simulink model "lqr_model"  (R2021a)
settings: Solver=VariableStepAuto  StartTime=0.0  StopTime=20  FixedStep=0.01  RelTol=1e-3
values from neighbouring files (symbols this model uses):
  FF_L = op.inputs(1).u    [trim_boat.m]
  initial_P = op.states(7).x    [trim_boat.m]
  initial_Q = op.states(3).x    [trim_boat.m]
  initial_R = op.states(8).x    [trim_boat.m]
  initial_uspeed = op.states(1).x    [trim_boat.m]
  initial_vspeed = op.states(6).x    [trim_boat.m]
  initial_wspeed = op.states(2).x    [trim_boat.m]
  initial_Z = op.states(5).x    [trim_boat.m]
  rear_alfas = op.inputs(3).u    [trim_boat.m]
  T = op.inputs(4).u    [trim_boat.m]
undefined symbols (not defined in the file or in its folder): ap2, ar2, ay2, bp2, br2, by2, Eff, K
libraries: simulink x4, pid_lib x1, dsparch4 x1
(part 1 of 2)
settings Model: Creator=Basile  LastModifiedBy=simao
settings SolverCC: ConcurrentTasks=on  ZeroCrossAlgorithm=Adaptive  AlgebraicLoopSolver=TrustRegion  PositivePriorityOrder=on
settings DataIOCC: ExternalInput=getinputstruct(op_trim1)  InitialState=getstatestruct(op_trim1)  SaveOutput=off  DSMLogging=off  SaveTime=off  ReturnWorkspaceOutputs=off
settings OptimizationCC: BlockReduction=off  DefaultParameterBehavior=Inlined  UseDivisionForNetSlopeComputation=on  UseFloatMulNetSlope=on  OptimizeBlockIOStorage=off  BufferReuse=off  PassReuseOutputArgsThreshold=0  EfficientFloat2IntCast=on  OptimizeBlockOrder=speed  DifferentSizesBufferReuse=on
settings DebuggingCC: InheritedTsInSrcMsg=none  ParameterTunabilityLossMsg=error  UnconnectedInputMsg=none  UnconnectedOutputMsg=none  UnconnectedLineMsg=none  UniqueDataStoreMsg=error  SFMachineParentedDataDiag=warning  ArithmeticOperatorsInVariantConditions=warning
settings HardwareCC: ProdBitPerLong=64  ProdLongLongMode=on  ProdHWDeviceType=Intel->x86-64 (Linux 64)
settings SFSimCC: SimUseLocalCustomCode=off  MATLABDynamicMemAlloc=off  CustomCodeUndefinedFunction=UseInterfaceOnly
settings RTWCC: Description=Simulink Real-Time  SystemTargetFile=slrealtime.tlc  TemplateMakefile=slrealtime_default_tmf  GenerateReport=on  RTWUseLocalCustomCode=off  Toolchain=Simulink Real-Time Toolchain  BuildConfiguration=Faster Runs  LaunchReport=on  CodeExecutionProfiling=on  TargetLang=C++
settings CodeAppCC: ForceParamTrailComments=on  OperatorAnnotations=on

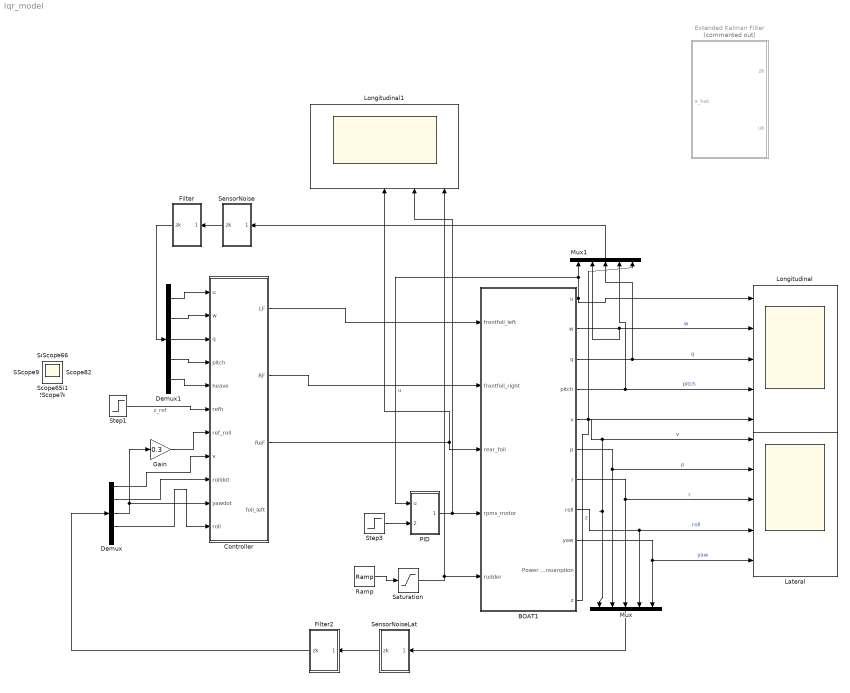
== system lqr_model ==
  BOAT1 : Subsystem
  Controller : Subsystem
  Demux : Demux  Outputs=5
  Demux1 : Demux  Outputs=5
  Extended Kalman Filter : Subsystem  Commented=on
  Filter : Subsystem
  Filter2 : Subsystem
  Gain : Gain  Gain=0.3
  Lateral : Scope  NumInputPorts=5
  Longitudinal : Scope  NumInputPorts=5
  Longitudinal1 : Scope  NumInputPorts=5
  Mux : Mux  Inputs=5
  Mux1 : Mux  Inputs=5
  PID : Subsystem
  Ramp : simulink/Sources/Ramp  slope=15  start=0  InitialOutput=0
  Saturation : Saturate  UpperLimit=0  LowerLimit=0
  SensorNoise : Subsystem
  SensorNoiseLat : Subsystem
  Step1 : Step  Time=0  Before=initial_Z  After=-0.4  SampleTime=0
  Step3 : Step  Time=0  Before=initial_uspeed  After=7  SampleTime=0
  Scope{,1..66} (67 alike) : Scope
  wires:
  BOAT1/2(w) -> Mux1/2, Longitudinal/2  "w"
  BOAT1/3(q) -> Mux1/3, Longitudinal/3  "q"
  BOAT1/5(v) -> Mux/1, Lateral/1  "v"
  BOAT1/6(p) -> Lateral/2, Mux/2  "p"
  BOAT1/8(roll) -> Lateral/4, Mux/4  "roll"
  BOAT1/11(z) -> Mux1/5, Longitudinal/5  "z"
  BOAT1/1(u) -> Longitudinal/1, PID/1(u), Mux1/1  "u"
  BOAT1/7(r) -> Lateral/3, Mux/3  "r"
  Demux1/2 -> Controller/2(w)
  Demux1/3 -> Controller/3(q)
  Demux1/4 -> Controller/4(pitch)
  Demux1/5 -> Controller/5(heave)
  Demux1/1 -> Controller/1(u)
  BOAT1/9(yaw) -> Mux/5, Lateral/5  "yaw"
  BOAT1/4(pitch) -> Mux1/4, Longitudinal/4  "pitch"
  Mux1/1 -> SensorNoise/1(states)
  Step1/1 -> Controller/6(refh)  "z_ref"
  Mux/1 -> SensorNoiseLat/1(states)
  Step3/1 -> PID/2(In2)
  Controller/3(ReF) -> BOAT1/3(rear_foil), Longitudinal1/3
  PID/1(rpms_motor) -> BOAT1/4(rpms_motor), Longitudinal1/4
  SensorNoise/1(zk) -> Filter/1(states)
  SensorNoiseLat/1(zk) -> Filter2/1(states)
  Filter/1(zk) -> Demux1/1
  Filter2/1(zk) -> Demux/1
  Gain/1 -> Controller/7(ref_roll)
  Ramp/1 -> Saturation/1
  Saturation/1 -> BOAT1/5(rudder), Longitudinal1/5
  Demux/2 -> Controller/9(rolldot)
  Demux/3 -> Gain/1, Controller/10(yawdot)
  Demux/4 -> Controller/11(roll)
  Demux/1 -> Controller/8(v)
  Controller/1(LF) -> BOAT1/1(frontfoil_left)
  Controller/2(RF) -> BOAT1/2(frontfoil_right)

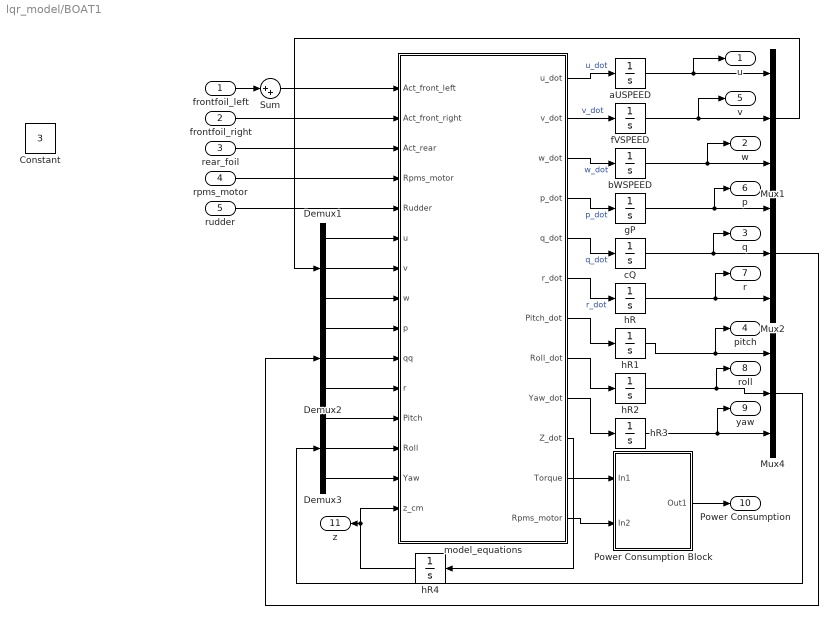
== system lqr_model/BOAT1 ==
  frontfoil_left : Inport
  frontfoil_right : Inport  Port=2
  rear_foil : Inport  Port=3
  rpms_motor : Inport  Port=4
  rudder : Inport  Port=5
  Constant : Constant  Value=3
  Demux1 : Demux  Outputs=3
  Demux2 : Demux  Outputs=3
  Demux3 : Demux  Outputs=3
  Mux1 : Mux  Inputs=3
  Mux2 : Mux  Inputs=3
  Mux4 : Mux  Inputs=3
  Power Consumption Block : Subsystem
  Sum : Sum  Inputs=|++
  aUSPEED : Integrator  InitialCondition=initial_uspeed
  bWSPEED : Integrator  InitialCondition=initial_wspeed
  cQ : Integrator  InitialCondition=initial_Q
  fVSPEED : Integrator  InitialCondition=initial_vspeed
  gP : Integrator  InitialCondition=initial_P
  hR : Integrator  InitialCondition=initial_R
  hR1 : Integrator
  hR2 : Integrator
  hR3 : Integrator
  hR4 : Integrator  InitialCondition=initial_Z
  model_equations : MATLAB Function  TreatAsAtomicUnit=on  VariantControl=Variant1
  u : Outport  VectorParamsAs1DForOutWhenUnconnected=off
  w : Outport  Port=2  VectorParamsAs1DForOutWhenUnconnected=off
  q : Outport  Port=3  VectorParamsAs1DForOutWhenUnconnected=off
  pitch : Outport  Port=4  VectorParamsAs1DForOutWhenUnconnected=off
  v : Outport  Port=5  VectorParamsAs1DForOutWhenUnconnected=off
  p : Outport  Port=6  VectorParamsAs1DForOutWhenUnconnected=off
  r : Outport  Port=7  VectorParamsAs1DForOutWhenUnconnected=off
  roll : Outport  Port=8  VectorParamsAs1DForOutWhenUnconnected=off
  yaw : Outport  Port=9  VectorParamsAs1DForOutWhenUnconnected=off
  Power Consumption : Outport  Port=10  VectorParamsAs1DForOutWhenUnconnected=off
  z : Outport  Port=11  VectorParamsAs1DForOutWhenUnconnected=off
  wires:
  model_equations/6(r_dot) -> hR/1  "r_dot"
  Mux1/1 -> Demux1/1
  model_equations/5(q_dot) -> cQ/1  "q_dot"
  rear_foil/1 -> model_equations/3(Act_rear)
  Demux3/2 -> model_equations/13(Roll)
  Demux2/2 -> model_equations/10(qq)
  Demux2/3 -> model_equations/11(r)
  model_equations/4(p_dot) -> gP/1  "p_dot"
  Demux2/1 -> model_equations/9(p)
  rpms_motor/1 -> model_equations/4("Rpms_motor ")
  Demux3/1 -> model_equations/12(Pitch)
  model_equations/2(v_dot) -> fVSPEED/1  "v_dot"
  Demux1/2 -> model_equations/7(v)
  Mux2/1 -> Demux2/1
  Demux3/3 -> model_equations/14(Yaw)
  model_equations/12(Rpms_motor) -> Power Consumption Block/2(In2)
  Power Consumption Block/1(Out1) -> Power Consumption/1
  model_equations/11(Torque) -> Power Consumption Block/1(In1)
  Demux1/1 -> model_equations/6(u)
  cQ/1 -> q/1, Mux2/2
  hR/1 -> Mux2/3, r/1
  model_equations/3(w_dot) -> bWSPEED/1  "w_dot"
  model_equations/1(u_dot) -> aUSPEED/1  "u_dot"
  gP/1 -> p/1, Mux2/1
  model_equations/7(Pitch_dot) -> hR1/1
  model_equations/8(Roll_dot) -> hR2/1
  model_equations/9(Yaw_dot) -> hR3/1
  hR1/1 -> pitch/1, Mux4/1
  hR2/1 -> roll/1, Mux4/2
  hR3/1 -> yaw/1, Mux4/3
  Mux4/1 -> Demux3/1
  rudder/1 -> model_equations/5(Rudder)
  frontfoil_right/1 -> model_equations/2(Act_front_right)
  frontfoil_left/1 -> Sum/1
  Sum/1 -> model_equations/1(Act_front_left)
  Demux1/3 -> model_equations/8(w)
  fVSPEED/1 -> v/1, Mux1/2
  aUSPEED/1 -> u/1, Mux1/1
  bWSPEED/1 -> w/1, Mux1/3
  model_equations/10(Z_dot) -> hR4/1
  hR4/1 -> model_equations/15(z_cm), z/1

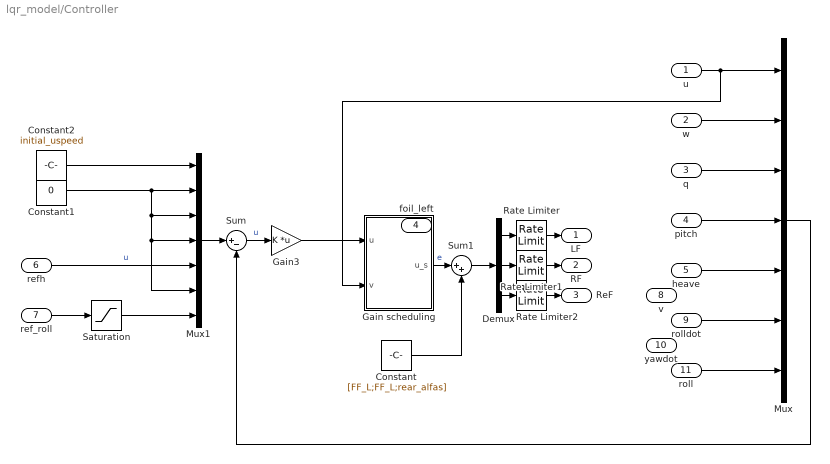
== system lqr_model/Controller ==
  u : Inport
  w : Inport  Port=2
  q : Inport  Port=3
  pitch : Inport  Port=4
  heave : Inport  Port=5
  refh : Inport  Port=6
  ref_roll : Inport  Port=7
  v : Inport  Port=8
  rolldot : Inport  Port=9
  yawdot : Inport  Port=10
  roll : Inport  Port=11
  Constant : Constant  Value=[FF_L;FF_L;rear_alfas]
  Constant1 : Constant  Value=0
  Constant2 : Constant  Value=initial_uspeed
  Demux : Demux  Outputs=3
  Gain scheduling : MATLAB Function  TreatAsAtomicUnit=on
  Gain3 : Gain  Gain=K  Multiplication=Matrix(K*u)
  Mux : Mux  Inputs=7
  Mux1 : Mux  Inputs=7
  Rate Limiter : RateLimiter  RisingSlewLimit=10  FallingSlewLimit=-10  SampleTimeMode=inherited  InitialCondition=FF_L
  Rate Limiter1 : RateLimiter  RisingSlewLimit=10  FallingSlewLimit=-10  SampleTimeMode=inherited  InitialCondition=FF_L
  Rate Limiter2 : RateLimiter  SampleTimeMode=inherited  InitialCondition=rear_alfas
  Saturation : Saturate  UpperLimit=3  LowerLimit=-3
  Sum : Sum  Inputs=|+-
  Sum1 : Sum  Inputs=|++
  LF : Outport  VectorParamsAs1DForOutWhenUnconnected=off
  RF : Outport  Port=2  VectorParamsAs1DForOutWhenUnconnected=off
  ReF : Outport  Port=3  VectorParamsAs1DForOutWhenUnconnected=off
  foil_left : Outport  Port=4  VectorParamsAs1DForOutWhenUnconnected=off
  wires:
  ref_roll/1 -> Saturation/1
  Mux/1 -> Sum/2
  u/1 -> Gain scheduling/2(v), Mux/1
  w/1 -> Mux/2
  q/1 -> Mux/3
  pitch/1 -> Mux/4
  heave/1 -> Mux/5
  rolldot/1 -> Mux/6
  roll/1 -> Mux/7
  Mux1/1 -> Sum/1
  refh/1 -> Mux1/5  "u"
  Sum/1 -> Gain3/1  "u"
  Saturation/1 -> Mux1/7
  Constant1/1 -> Mux1/6, Mux1/4, Mux1/3, Mux1/2
  Constant2/1 -> Mux1/1
  Gain3/1 -> Gain scheduling/1(u)
  Gain scheduling/1(u_s) -> Sum1/1  "e"
  Sum1/1 -> Demux/1
  Constant/1 -> Sum1/2
  Demux/1 -> Rate Limiter/1
  Rate Limiter/1 -> LF/1
  Demux/2 -> Rate Limiter1/1
  Rate Limiter1/1 -> RF/1
  Demux/3 -> Rate Limiter2/1
  Rate Limiter2/1 -> ReF/1

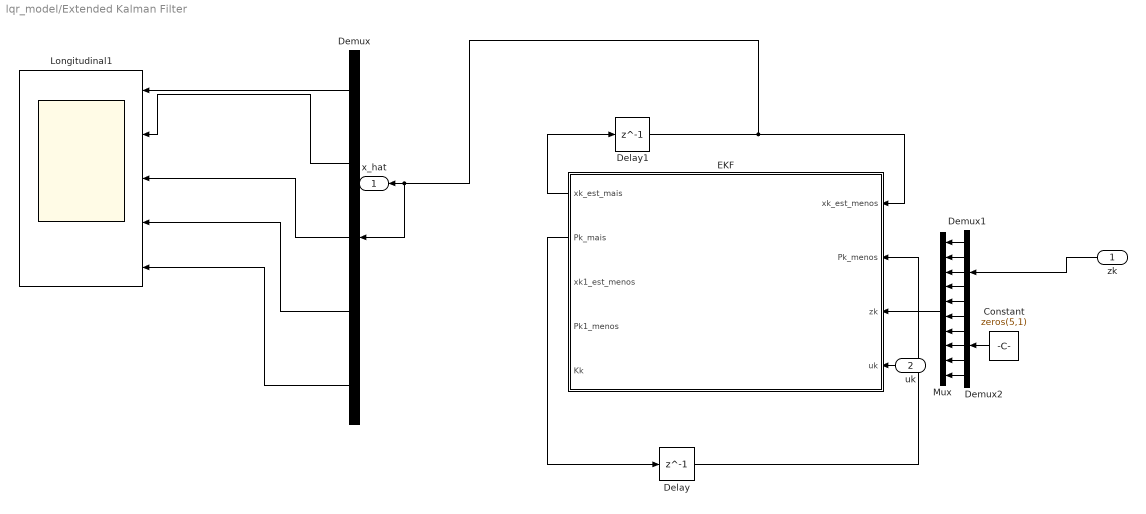
== system lqr_model/Extended Kalman Filter ==
  zk : Inport  PortDimensions=5
  uk : Inport  Port=2  PortDimensions=5
  Constant : Constant  Value=zeros(5,1)
  Delay : Delay  DelayLength=1  InitialCondition=1000*eye(37)  SampleTime=0.02
  Delay1 : Delay  DelayLength=1  InitialCondition=[initial_uspeed;0;0;0;initial_Z;0;0;0;0;0;zeros(27,1)]  SampleTime=0.02
  Demux : Demux  Outputs=5
  Demux1 : Demux  Outputs=5
  Demux2 : Demux  Outputs=5
  EKF : MATLAB Function  TreatAsAtomicUnit=on
  Longitudinal1 : Scope  NumInputPorts=5
  Mux : Mux  Inputs=10
  x_hat : Outport
  wires:
  uk/1 -> EKF/4(uk)
  Delay/1 -> EKF/2(Pk_menos)
  Demux/1 -> Longitudinal1/1
  Demux/2 -> Longitudinal1/2
  Demux/3 -> Longitudinal1/3
  Demux/4 -> Longitudinal1/4
  Demux/5 -> Longitudinal1/5
  Delay1/1 -> Demux/1, x_hat/1, EKF/1(xk_est_menos)
  EKF/2(Pk_mais) -> Delay/1
  EKF/1(xk_est_mais) -> Delay1/1
  zk/1 -> Demux1/1
  Mux/1 -> EKF/3(zk)
  Demux1/1 -> Mux/1
  Demux1/2 -> Mux/2
  Demux1/3 -> Mux/3
  Demux1/4 -> Mux/4
  Demux1/5 -> Mux/5
  Demux2/1 -> Mux/6
  Demux2/2 -> Mux/7
  Demux2/3 -> Mux/8
  Demux2/4 -> Mux/9
  Demux2/5 -> Mux/10
  Constant/1 -> Demux2/1

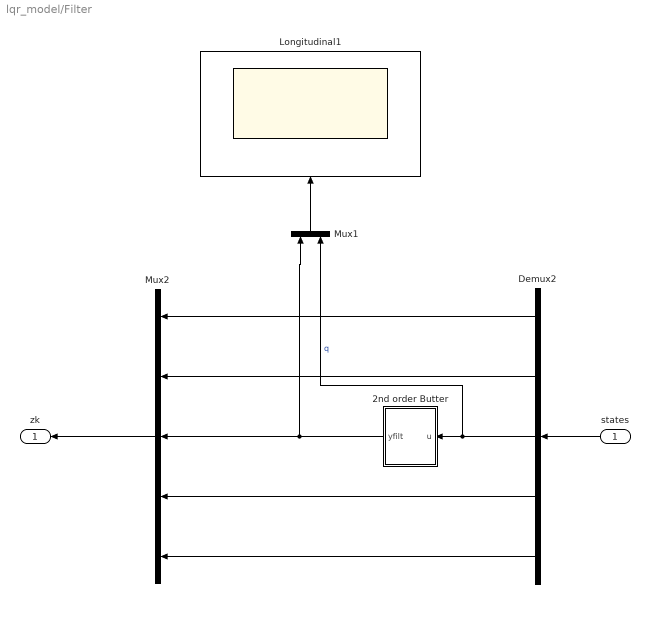
== system lqr_model/Filter ==
  states : Inport
  2nd order Butter : Subsystem
  Demux2 : Demux  Outputs=5
  Longitudinal1 : Scope  NumInputPorts=5
  Mux1 : Mux  Inputs=2
  Mux2 : Mux  Inputs=5
  zk : Outport
  wires:
  states/1 -> Demux2/1
  Mux2/1 -> zk/1
  Demux2/1 -> Mux2/1
  Demux2/2 -> Mux2/2
  Demux2/4 -> Mux2/4
  Demux2/5 -> Mux2/5
  Mux1/1 -> Longitudinal1/3
  2nd order Butter/1(yfilt) -> Mux1/1, Mux2/3
  Demux2/3 -> Mux1/2, 2nd order Butter/1(u)  "q"

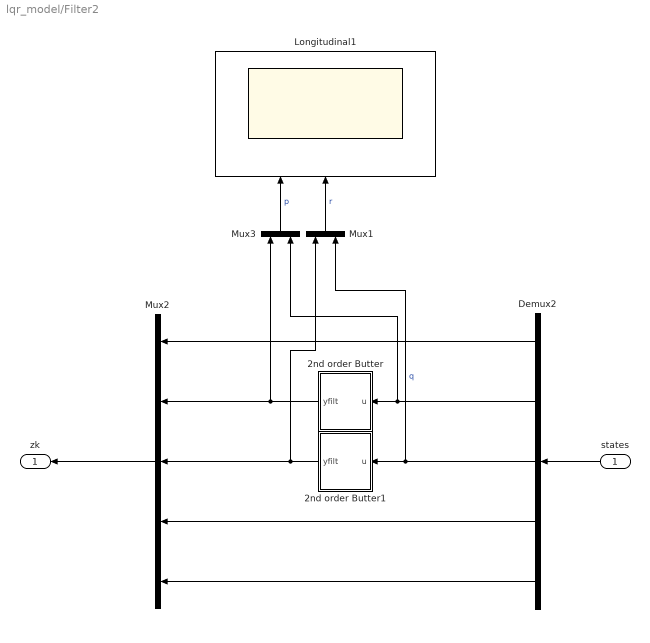
== system lqr_model/Filter2 ==
  states : Inport
  2nd order Butter : Subsystem
  2nd order Butter1 : Subsystem
  Demux2 : Demux  Outputs=5
  Longitudinal1 : Scope  NumInputPorts=5
  Mux1 : Mux  Inputs=2
  Mux2 : Mux  Inputs=5
  Mux3 : Mux  Inputs=2
  zk : Outport
  wires:
  states/1 -> Demux2/1
  Mux2/1 -> zk/1
  Demux2/1 -> Mux2/1
  Demux2/4 -> Mux2/4
  Demux2/5 -> Mux2/5
  Demux2/2 -> Mux3/2, 2nd order Butter/1(u)
  2nd order Butter/1(yfilt) -> Mux3/1, Mux2/2
  2nd order Butter1/1(yfilt) -> Mux1/1, Mux2/3
  Demux2/3 -> Mux1/2, 2nd order Butter1/1(u)  "q"
  Mux1/1 -> Longitudinal1/3  "r"
  Mux3/1 -> Longitudinal1/2  "p"

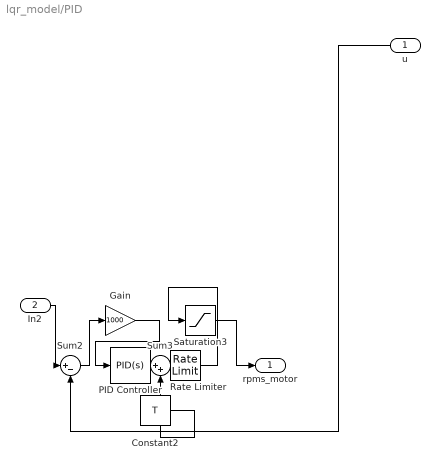
== system lqr_model/PID ==
  u : Inport
  In2 : Inport  Port=2
  Constant2 : Constant  Value=T
  Gain : Gain  Gain=1000
  PID Controller : pid_lib/PID Controller  Controller=PID  Form=Parallel  TimeDomain=Continuous-time  UseExternalTs=off  SampleTime=-1  IntegratorMethod=Forward Euler  FilterMethod=Forward Euler  ControllerParametersSource=internal  P=1  I=1  D=0.00001  UseFilter=on  N=100  TunerSelectOption=Transfer Function Based (PID Tuner App)  InitialConditionSource=internal  InitialConditionForIntegrator=0  InitialConditionForFilter=0  DifferentiatorICPrevScaledInput=0  ExternalReset=none  TrackingMode=off  Kt=1  LimitOutput=off  SatLimitsSource=internal  UpperSaturationLimit=inf  LowerSaturationLimit=-inf  LinearizeAsGain=on  AntiWindupMode=none  Kb=1  POutMin=[]  POutMax=[]  IOutMin=[]  IOutMax=[]  DOutMin=[]  DOutMax=[]  NOutMin=[]  NOutMax=[]  SumOutMin=[]  SumOutMax=[]  SaturationOutMin=[]  SaturationOutMax=[]  PParamMin=[]  PParamMax=[]  IParamMin=[]  IParamMax=[]  DParamMin=[]  DParamMax=[]  NParamMin=[]  NParamMax=[]  KbParamMin=[]  KbParamMax=[]  KtParamMin=[]  KtParamMax=[]  KbOutMin=[]  KbOutMax=[]  KtOutMin=[]  KtOutMax=[]  IntegratorOutMin=[]  IntegratorOutMax=[]  FilterOutMin=[]  FilterOutMax=[]  SumI1OutMin=[]  SumI1OutMax=[]  SumI2OutMin=[]  SumI2OutMax=[]  SumI3OutMin=[]  SumI3OutMax=[]  SumI4OutMin=[]  SumI4OutMax=[]  SumDOutMin=[]  SumDOutMax=[]  DifferentiatorOutMin=[]  DifferentiatorOutMax=[]  FilterDiffOutCoefMin=[]  FilterDiffOutCoefMax=[]  ReciprocalOutMin=[]  ReciprocalOutMax=[]  SumDenOutMin=[]  SumDenOutMax=[]  SumNumOutMin=[]  SumNumOutMax=[]  DivideOutMin=[]  DivideOutMax=[]  UdiffTsProdOutMin=[]  UdiffTsProdOutMax=[]  NTsProdOutMin=[]  NTsProdOutMax=[]  UintegralTsProdOutMin=[]  UintegralTsProdOutMax=[]  UngainTsProdOutMin=[]  UngainTsProdOutMax=[]  IntegratorContinuousStateAttributes=''  IntegratorStateMustResolveToSignalObject=off  IntegratorRTWStateStorageClass=Auto  FilterContinuousStateAttributes=''  FilterStateMustResolveToSignalObject=off  FilterRTWStateStorageClass=Auto  ParallelPVariant=InternalParameters  IdealPVariant=Disabled  IVariant=InternalParameters  DVariant=InternalParameters  IntegratorVariant=Continuous  SatVariant=Disabled  AWVariant=Passthrough  PCopyVariant=Disabled  TRVariant=Disabled  FdbkBlocksVariant=Forward  IdealPFdbkVariant=Disabled  SatFdbkVariant=Disabled  DerivativeFilterVariant=ContFilter  NVariant=InternalParameters  NCopyVariant=Disabled  FilterICVariant=InternalICsFilter  IntegratorICVariant=InternalICs  ExternalResetVariant=Disabled  TRSumVariant=Passthrough  SumFdbkVariant=Disabled  SumVariant=Sum_PID  TsampFilterVariant=InternalTs  TsampNgainVariant=Passthrough  TsampIntegralVariant=Passthrough  ExternalSaturationOutDataTypeStr=Inherit: Same as second input
  Rate Limiter : RateLimiter  RisingSlewLimit=1000  FallingSlewLimit=-1000  SampleTimeMode=inherited  InitialCondition=T
  Saturation3 : Saturate  UpperLimit=9000
  Sum2 : Sum  Inputs=|+-
  Sum3 : Sum  Inputs=|++
  rpms_motor : Outport
  wires:
  u/1 -> Sum2/2
  Sum3/1 -> Rate Limiter/1
  Gain/1 -> PID Controller/1
  Saturation3/1 -> rpms_motor/1
  PID Controller/1 -> Sum3/1
  Rate Limiter/1 -> Saturation3/1
  Sum2/1 -> Gain/1
  In2/1 -> Sum2/1
  Constant2/1 -> Sum3/2

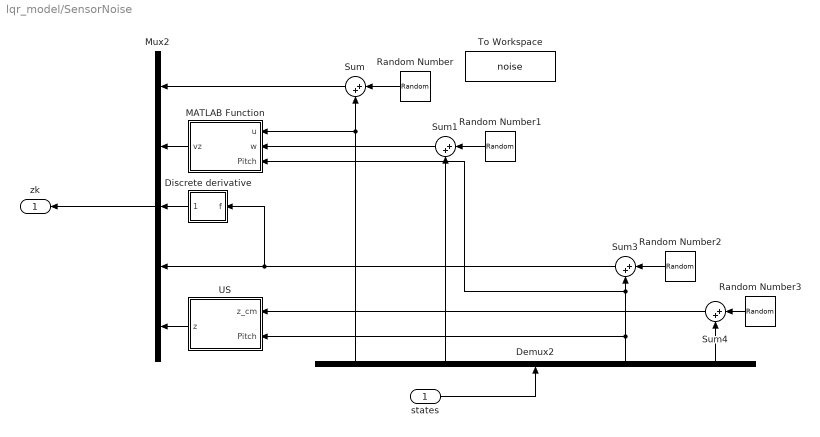
== system lqr_model/SensorNoise ==
  states : Inport
  Demux2 : Demux  Outputs=5
  Discrete derivative : Subsystem
  MATLAB Function : MATLAB Function  TreatAsAtomicUnit=on
  Mux2 : Mux  Inputs=5
  Random Number : RandomNumber  Variance=0.001^2  Seed=31233  SampleTime=0.02
  Random Number1 : RandomNumber  Variance=0.001^2  Seed=31232  SampleTime=0.02
  Random Number2 : RandomNumber  Variance=0.005^2  Seed=372323  SampleTime=0.02
  Random Number3 : RandomNumber  Variance=0.0005^2  Seed=312392  SampleTime=0.02
  Sum{,1,3..4} (4 alike) : Sum  Inputs=|++
  To Workspace : ToWorkspace  VariableName=noise  SaveFormat=Timeseries  SampleTime=0.02
  US : MATLAB Function  TreatAsAtomicUnit=on
  zk : Outport
  wires:
  Demux2/1 -> MATLAB Function/1(u), Sum/2
  Random Number2/1 -> Sum3/1
  Random Number3/1 -> Sum4/1
  Random Number/1 -> Sum/1
  Demux2/4 -> MATLAB Function/3(Pitch), Sum3/2, US/2(Pitch)
  Demux2/5 -> Sum4/2
  Demux2/2 -> Sum1/2
  Random Number1/1 -> Sum1/1
  states/1 -> Demux2/1
  Mux2/1 -> zk/1
  Sum/1 -> Mux2/1
  Sum3/1 -> Discrete derivative/1(f), Mux2/4
  US/1(z) -> Mux2/5
  Sum4/1 -> US/1(z_cm)
  Sum1/1 -> MATLAB Function/2(w)
  MATLAB Function/1(vz) -> Mux2/2
  Discrete derivative/1(fdot) -> Mux2/3

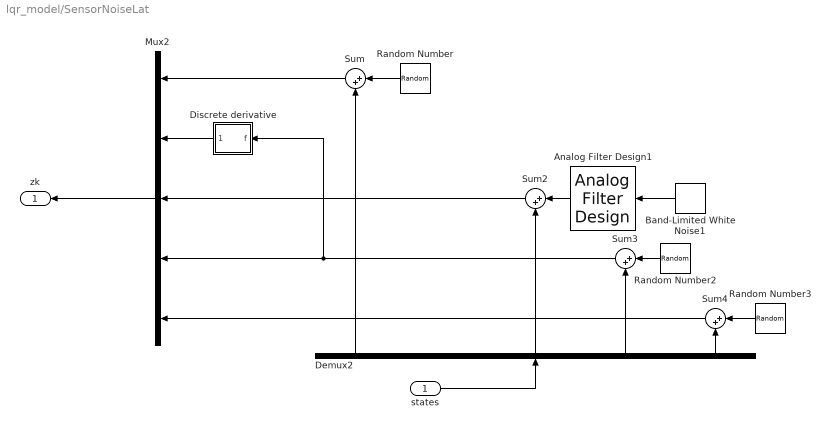
== system lqr_model/SensorNoiseLat ==
  states : Inport
  Analog Filter Design1 : dsparch4/Analog Filter Design  method=Butterworth  filttype=Highpass  N=8  Wlo=3*2*pi  Whi=80  Rp=2  Rs=40
  Band-Limited White Noise1 : simulink/Sources/Band-Limited White Noise  Cov=[0.00005]  Ts=0.02  seed=[23341]
  Demux2 : Demux  Outputs=5
  Discrete derivative : Subsystem
  Mux2 : Mux  Inputs=5
  Random Number : RandomNumber  Variance=0.05^2  Seed=31233  SampleTime=0.02
  Random Number2 : RandomNumber  Variance=0.005^2  Seed=372323  SampleTime=0.02
  Random Number3 : RandomNumber  Variance=0.005^2  Seed=312392  SampleTime=0.02
  Sum{,2..4} (4 alike) : Sum  Inputs=|++
  zk : Outport
  wires:
  Demux2/1 -> Sum/2
  Random Number2/1 -> Sum3/1
  Random Number3/1 -> Sum4/1
  Random Number/1 -> Sum/1
  Demux2/4 -> Sum3/2
  Demux2/3 -> Sum2/2
  Demux2/5 -> Sum4/2
  states/1 -> Demux2/1
  Mux2/1 -> zk/1
  Sum/1 -> Mux2/1
  Sum2/1 -> Mux2/3
  Sum3/1 -> Discrete derivative/1(f), Mux2/4
  Sum4/1 -> Mux2/5
  Band-Limited White Noise1/1 -> Analog Filter Design1/1
  Analog Filter Design1/1 -> Sum2/1
  Discrete derivative/1(fdot) -> Mux2/2

== system lqr_model/BOAT1/Power Consumption Block ==
  In1 : Inport
  In2 : Inport  Port=2
  2-D Lookup Table : Lookup_n-D  BreakpointsForDimension1=[1:6000]  BreakpointsForDimension2=[1:140]  Table=Eff  InternalRulePriority=Speed  RndMeth=Simplest  InputSameDT=on
      settings: InputPortMap=u0,u1
  Gain : Gain  Gain=10
  MATLAB Function1 : MATLAB Function  TreatAsAtomicUnit=on
  Out1 : Outport
  wires:
  In2/1 -> 2-D Lookup Table/1, MATLAB Function1/2(Rpms_motor)
  MATLAB Function1/1(P_elec) -> Out1/1
  In1/1 -> Gain/1, MATLAB Function1/1(Torque)
  Gain/1 -> 2-D Lookup Table/2
  2-D Lookup Table/1 -> MATLAB Function1/3(Eficiencia_motor)

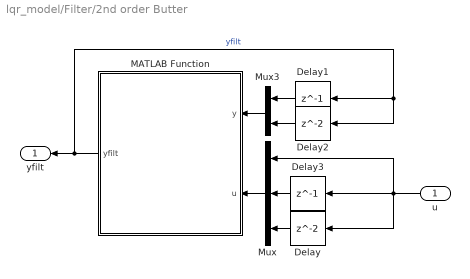
== system lqr_model/Filter/2nd order Butter ==
  u : Inport
  Delay : Delay
  Delay1 : Delay  DelayLength=1  SampleTime=0.02
  Delay2 : Delay
  Delay3 : Delay  DelayLength=1  SampleTime=0.02
  MATLAB Function : MATLAB Function  TreatAsAtomicUnit=on
  Mux : Mux  Inputs=3
  Mux3 : Mux  Inputs=2
  yfilt : Outport
  wires:
  Mux3/1 -> MATLAB Function/1(y)
  Mux/1 -> MATLAB Function/2(u)
  MATLAB Function/1(yfilt) -> Delay1/1, Delay2/1, yfilt/1  "yfilt"
  Delay/1 -> Mux/3
  Delay3/1 -> Mux/2
  u/1 -> Mux/1, Delay3/1, Delay/1
  Delay1/1 -> Mux3/1
  Delay2/1 -> Mux3/2

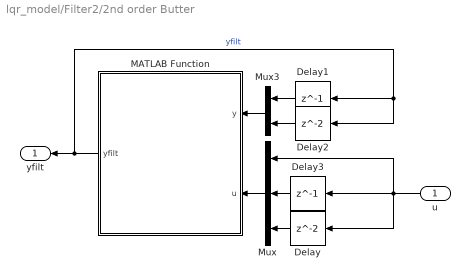
== system lqr_model/Filter2/2nd order Butter ==
  u : Inport
  Delay : Delay
  Delay1 : Delay  DelayLength=1  SampleTime=0.02
  Delay2 : Delay
  Delay3 : Delay  DelayLength=1  SampleTime=0.02
  MATLAB Function : MATLAB Function  TreatAsAtomicUnit=on
  Mux : Mux  Inputs=3
  Mux3 : Mux  Inputs=2
  yfilt : Outport
  wires:
  Mux3/1 -> MATLAB Function/1(y)
  Mux/1 -> MATLAB Function/2(u)
  MATLAB Function/1(yfilt) -> Delay1/1, Delay2/1, yfilt/1  "yfilt"
  Delay/1 -> Mux/3
  Delay3/1 -> Mux/2
  u/1 -> Mux/1, Delay3/1, Delay/1
  Delay1/1 -> Mux3/1
  Delay2/1 -> Mux3/2

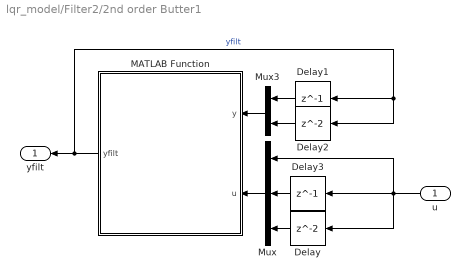
== system lqr_model/Filter2/2nd order Butter1 ==
  u : Inport
  Delay : Delay
  Delay1 : Delay  DelayLength=1  SampleTime=0.02
  Delay2 : Delay
  Delay3 : Delay  DelayLength=1  SampleTime=0.02
  MATLAB Function : MATLAB Function  TreatAsAtomicUnit=on
  Mux : Mux  Inputs=3
  Mux3 : Mux  Inputs=2
  yfilt : Outport
  wires:
  Mux3/1 -> MATLAB Function/1(y)
  Mux/1 -> MATLAB Function/2(u)
  MATLAB Function/1(yfilt) -> Delay1/1, Delay2/1, yfilt/1  "yfilt"
  Delay/1 -> Mux/3
  Delay3/1 -> Mux/2
  u/1 -> Mux/1, Delay3/1, Delay/1
  Delay1/1 -> Mux3/1
  Delay2/1 -> Mux3/2

== system lqr_model/SensorNoise/Discrete derivative ==
  f : Inport
  Constant : Constant  Value=0
  Discrete Derivative : simulink/Discrete/Discrete Derivative  gainval=1.0  ICPrevScaledInput=0.0  OutMin=[]  OutMax=[]  OutDataType=fixdt(1, 16)  OutScaling=2^-10  DoSatur=off
  Step : Step  Time=0.01  Before=-1
  Switch : Switch  Criteria=u2 > Threshold
  fdot : Outport  VectorParamsAs1DForOutWhenUnconnected=off
  wires:
  Discrete Derivative/1 -> Switch/1  "ddtkz"
  Constant/1 -> Switch/3
  Step/1 -> Switch/2
  f/1 -> Discrete Derivative/1
  Switch/1 -> fdot/1

== system lqr_model/SensorNoiseLat/Discrete derivative ==
  f : Inport
  Constant : Constant  Value=0
  Discrete Derivative : simulink/Discrete/Discrete Derivative  gainval=1.0  ICPrevScaledInput=0.0  OutMin=[]  OutMax=[]  OutDataType=fixdt(1, 16)  OutScaling=2^-10  DoSatur=off
  Step : Step  Time=0.01  Before=-1
  Switch : Switch  Criteria=u2 > Threshold
  fdot : Outport  VectorParamsAs1DForOutWhenUnconnected=off
  wires:
  Discrete Derivative/1 -> Switch/1  "ddtkz"
  Constant/1 -> Switch/3
  Step/1 -> Switch/2
  f/1 -> Discrete Derivative/1
  Switch/1 -> fdot/1

== matlab function lqr_model/Controller/Gain scheduling ==
  data: u input; u_s output; v input
function u_s = fcn(u,v)
v_ref = 7;
if(v>v_ref)
    u_s = u*v_ref^2/v^2;
else
    u_s = u;
end

== matlab function lqr_model/SensorNoise/US ==
  data: z_cm input; z output; Pitch input
function z = fcn(z_cm,Pitch)
Roll = 0; %Approximation
dist_cm_Us_x = 3.150;   %distance between cm and US
z = (z_cm*cosd(Roll)-tand(Pitch)*dist_cm_Us_x)/cosd(Pitch);

== matlab function lqr_model/Filter/2nd order Butter/MATLAB Function ==
  data: y input; u input; yfilt output; bp2 parameter; ap2 parameter
function yfilt = filtit(y,u, bp2, ap2)
b = bp2;
a = ap2;
yfilt = 0;
for i=1:length(u)
   yfilt = yfilt + b(i)*u(i);
end

for i=2:length(y)+1
   yfilt = yfilt - a(i)*y(i-1); 
end

yfilt = yfilt/a(1);

end

== matlab function lqr_model/Filter2/2nd order Butter/MATLAB Function ==
  data: y input; u input; yfilt output; br2 parameter; ar2 parameter
function yfilt = filtit(y,u, br2, ar2)
b = br2;
a = ar2;
yfilt = 0;
for i=1:length(u)
   yfilt = yfilt + b(i)*u(i);
end

for i=2:length(y)+1
   yfilt = yfilt - a(i)*y(i-1); 
end

yfilt = yfilt/a(1);

end

== matlab function lqr_model/Extended Kalman Filter/EKF ==
  data: xk_est_mais output; xk_est_menos input; Pk_menos input; zk input; Pk_mais output; xk1_est_menos output; Pk1_menos output; Kk output; uk input
function [xk_est_mais,Pk_mais,xk1_est_menos,Pk1_menos,Kk] = extended_kalman_filter(xk_est_menos,Pk_menos,zk,uk)

%EKF matrices
Rk = diag([0.05^2 0.05^2 0.25^2 0.25^2 0.005^2 0 0 0 0 0]); 
Qku = eye(10); %Quando tiver erro de modelo

%% RKM Aproximation

%Prediction Phase
%Phik = Jacobian_func_out(xk_est_menos(1),xk_est_menos(2),xk_est_menos(3),xk_est_menos(4),xk_est_menos(5),xk_est_menos(6),xk_est_menos(7),xk_est_menos(8),xk_est_menos(9),uk(3),uk(2),uk(1),uk(4),uk(5));
Phik = fwjac(xk,uk);
Phik = expm(Phik*0.02);
Qk = Phik*Qku*Phik'*0.02;
xk1_est_menos = RKM_EKF(xk_est_menos,uk);
Pk1_menos = Phik*Pk_menos*Phik'+Qk;

%Correction Phase
yk = xk1_est_menos;
Hk = Hk_func(xk1_est_menos(4),xk1_est_menos(5),xk1_est_menos(9));
yk(5) = (yk(5)*cosd(yk(9))-tand(yk(4))*dist_cm_Us_x)/cosd(yk(4)); 
Kk = Pk1_menos*Hk'*inv(Hk*Pk1_menos*Hk'+Rk);
xk_est_mais = xk1_est_menos+Kk*(zk-yk);
Pk_mais = (eye(10)-Kk*Hk)*Pk1_menos*(eye(10)-Kk*Hk)'+Kk*Rk*Kk';
end

== matlab function lqr_model/BOAT1/Power Consumption Block/MATLAB Function1 ==
  data: Torque input; P_elec output; Rpms_motor input; Eficiencia_motor input
function P_elec = fcn(Torque,Rpms_motor,Eficiencia_motor)
P_mec = Torque*Rpms_motor*2*pi/60;
P_elec = P_mec/Eficiencia_motor;

== matlab function lqr_model/BOAT1/model_equations ==
  data: u_dot output; v_dot output; w_dot output; p_dot output; q_dot output; r_dot output; Pitch_dot output; Roll_dot output; Yaw_dot output; Z_dot output; Act_front_left input; Act_front_right input; Act_rear input; Rpms_motor input; Rudder input; u input; v input; w input; p input; qq input; r input; Pitch input; Roll input; Yaw input; Torque output; Rpms_motor output; z_cm input
function [u_dot,v_dot,w_dot,p_dot,q_dot,r_dot,Pitch_dot,Roll_dot,Yaw_dot,Z_dot,Torque,Rpms_motor] = model_equations(Act_front_left,Act_front_right,Act_rear,Rpms_motor,Rudder,u,v,w,p,qq,r,Pitch,Roll,Yaw,z_cm)

%%%%%%%%%%%%%%%%%%%%%%%%%%%%%%%%%%%%%%%%%%%%%%%%%SS
%%%%%%%%%%%%%%%% constants %%%%%%%%%%%%%%%%%%%%%%
%%%%%%%%%%%%%%%%%%%%%%%%%%%%%%%%%%%%%%%%%%%%%%%%%
g = 9.81; %gravity (m/s^2)
rho= 1025.00; % Water density(kg/m^3)   <-I
mu= 1.14E-3; % Coef. Viscosidade Dinâmica para calular Reynolds(Pa*s)   <-I
m = 180; %Weight of boat (Kg) <-I
dist_cm_Us_x = 3.150;   %distance between cm and US in the x axis
dist_S_Us_x = 1.850;  %distance from struts to US in the x axis
dist_S_cm_x = 1.3;  %distance from struts to cm in the x axis
dist_C_Us_x = 5.520;  %distance from column to US in the x axis
dist_FF_cm_y = 1.2/2; %front foils' y distance divided by 2
dist_C_cm_x = 2.367; %distance from the column to cm in the x axis
dist_FF_cm_x = 1.30156; %distance from the front foils to cm in the x axis
dist_ReF_cm_z = 1.05; %distance from the rear foil to cm in the z axis
dist_FF_cm_z = 0.85; %distance from the front foils to cm in the z axis

% Height at each point 
z = (z_cm*cosd(Roll)-tand(Pitch)*dist_cm_Us_x)/cosd(Pitch);  %distance at US
z_S_no_roll = z+dist_S_Us_x*tand(Pitch); %Perpendicular distance to water of the struts 
z_C_no_roll = z+dist_C_Us_x*tand(Pitch); %Perpendicular distance to water of the column
z_LS = z_S_no_roll - tand(Roll)*dist_FF_cm_y; %Accounting for Roll
z_RS = z_S_no_roll + tand(Roll)*dist_FF_cm_y; %Accounting for Roll

% Depth of struts and column
h_LS = dist_FF_cm_z + z_LS;  
h_RS = dist_FF_cm_z + z_RS;
h_C = dist_ReF_cm_z + z_C_no_roll;

Iyy = 503;        % boat's moment of inertia in kg.m^2 for pitch
Ixx = 31;         % moment of inertia in kg.m^2 for roll
Izz = 300;        % boat's moment of inertia in kg.m^2 for yaw
Ixz = 16.5;       % boat's moment of inertia in kg.m^2 for roll/yaw

%strut and column lift center depende on heave
C_CoP = h_C/2 - z_C_no_roll; %column center of pressure
LS_CoP = h_LS/2 - z_LS; %Left strut center of pressure
RS_CoP = h_RS/2 - z_RS; %Right strut center of pressure

ww = [p;qq;r];
%Inertial angular velocities
Q = [1 sind(Roll)*tand(Pitch) cosd(Roll)*tand(Pitch);
     0 cosd(Roll) -sind(Roll);
     0 sind(Roll)/cosd(Pitch) cosd(Roll)/cosd(Pitch)];
eul = Q*ww;
Roll_dot = eul(1);
Pitch_dot = eul(2);
Yaw_dot = eul(3);
W = pi/180*[Roll_dot;Pitch_dot;Yaw_dot];

%Inertial to body frame matrix
R = [cosd(Pitch)*cosd(Yaw) cosd(Pitch)*sind(Yaw) -sind(Pitch);
    sind(Roll)*sind(Pitch)*cosd(Yaw)-cosd(Roll)*sind(Yaw) sind(Roll)*sind(Pitch)*sind(Yaw)+cosd(Roll)*cosd(Yaw) sind(Roll)*cosd(Pitch);
    cosd(Roll)*sind(Pitch)*cosd(Yaw)+sind(Roll)*sind(Yaw) cosd(Roll)*sind(Pitch)*sind(Yaw)-sind(Roll)*cosd(Yaw) cosd(Roll)*cosd(Pitch)];

%speed at each point - rotational kinematics Vp = Vo + WxRp
%Left strut
R_LS = [dist_S_cm_x;-dist_FF_cm_y;LS_CoP];
V_LS = [u;v;w] + cross(W,R_LS);
%Right Strut
R_RS = [dist_S_cm_x;dist_FF_cm_y;RS_CoP];
V_RS = [u;v;w] + cross(W,R_RS);
%Column
R_C = [-dist_C_cm_x;0;C_CoP];
V_C = [u;v;w] + cross(W,R_C);
%Left foil
R_LF = [dist_S_cm_x;-dist_FF_cm_y;dist_FF_cm_z];
V_LF = [u;v;w] + cross(W,R_LF);
%Right foil
R_RF = [dist_S_cm_x;dist_FF_cm_y;dist_FF_cm_z];
V_RF = [u;v;w] + cross(W,R_RF);
%Rear foil
R_RE = [-dist_C_cm_x;0;dist_ReF_cm_z];
V_ReF = [u;v;w] + cross(W,R_RE);

%angle of attack at each point
bb_C = asind(V_C(2)/V_C(1));
bb_LS = atand(V_LS(2)/V_LS(1));
bb_RS = atand(V_RS(2)/V_RS(1));
aa_LF = atand(V_LF(3)/V_LF(1));
aa_RF = atand(V_RF(3)/V_RF(1));
aa_ReF = atand(V_ReF(3)/V_ReF(1));
eff_aa_LF = Act_front_left + aa_LF;
eff_aa_RF = Act_front_right + aa_RF;
eff_aa_ReF = Act_rear + aa_ReF;

%Speed vector's magnitude at each point
speed_cm = sqrt(u^2+v^2+w^2); 
speed_LF = norm(V_LF);
speed_RF = norm(V_RF);
speed_ReF = norm(V_ReF);
speed_C = norm(V_C);
speed_LS = norm(V_LS);
speed_RS = norm(V_RS);

%Dynamic pressure at each point
q_LF = 0.5*rho*speed_LF^2;
q_RF = 0.5*rho*speed_RF^2;
q_ReF = 0.5*rho*speed_ReF^2;
q_C = 0.5*rho*speed_C^2;
q_LS = 0.5*rho*speed_LS^2;
q_RS = 0.5*rho*speed_RS^2;

%Geometria foil frente(x2)
c_FF=0.08; % Corda foil frente(m)
t_FF=0.12; % Espessura maxima perfil foil frente (n63412: t=0.12c)
b_FF=0.82; % Envergadura foil frente (m)
S_FF=pi*b_FF*c_FF/4; %Area planform foil frente (m^2) --  0.04773 valor dos foils atuais
SA_FF=S_FF*2; % Area superficie foil frente (assumir 2x planform area) (m^2)
AR_FF=b_FF^2/S_FF; %Aspect ratio foil frente
cordfun = @(x) c_FF.^2 .*(x-(x.^3/(b_FF/2).^2)/3);
MAC_FF =  2/S_FF*(cordfun(b_FF/2)-cordfun(0));
c_FF=MAC_FF; %Chord according to MAC
k2_LF = (16*(h_LS/MAC_FF)^2+2)/(16*(h_LS/MAC_FF)^2+1);
k2_RF = (16*(h_RS/MAC_FF)^2+2)/(16*(h_RS/MAC_FF)^2+1);
T_FF=c_FF*t_FF; % Thickness front foil= chord*t

CM_ac= -0.195; %valor para a asa do 02; a variação no intervalo de velocidades [6;8] m/s é desprezável. Posssibilidade de introduzir uma função que estima este paraâmetro através de outros (cenas de EVoo)
 %o valor usado para o calculo do momento é das quantidades locais na
 %respetiva asa 


%Geometria foil trás
c_ReF=0.08; % Corda foil trás (m)
t_ReF=0.12; % Espessura maxima foil tras (n63412: t=0.12c)
b_ReF=0.82; % Envergadura foil tras (m)
S_ReF=pi*b_ReF*c_ReF/4; %Area planform foil tras (m^2) --- 0.04584 valor dos foils atuais
SA_ReF=S_ReF*2; % Area superficie foil tras (assumir 2x planform area) (m^2)
AR_ReF=b_ReF^2/S_ReF; %Aspect ratio foil tras
cordfun = @(x) c_ReF.^2 .*(x-(x.^3/(b_ReF/2).^2)/3);
MAC_ReF = 2/S_ReF*(cordfun(b_ReF/2)-cordfun(0));
c_ReF=MAC_ReF; %Chord according to MAC
k2_ReF = (16*(h_C/MAC_ReF)^2+2)/(16*(h_C/MAC_FF)^2+1);
T_ReF=c_ReF*t_ReF;% Thickness rear foil= chord*t


%Struts geometry
c_S= 0.13; % Corda strut (m)
t_S=0.12; % Espessura maxima perfil strut (n0012: t=0.12c)
T_S=c_S*t_S; % Thickness strut= chord*t
%Left Strut
S_LS=c_S*h_LS; %area planform strut (m^2)
SA_LS=2*S_LS; % Area superficie strut (SOLIDWORKS) (m^2)
sub_LS=h_LS/c_S; %aspect ratio da seccao submergida strut
%Right Strut
S_RS=c_S*h_RS; %area planform strut (m^2)
SA_RS=2*S_RS; % Area superficie strut (SOLIDWORKS) (m^2)
sub_RS=h_RS/c_S; %aspect ratio da seccao submergida strut

%Column geometry
c_C=0.17; % corda coluna (m)
t_C=0.18; % Espessura maxima perfil coluna (n0012: t=0.12c)
S_C=c_C*h_C; %area planform coluna (m^2)
SA_C=2*S_C; % Area superficie coluna (m^2)
sub_C=h_C/c_C; %aspect ratio da seccao submergida coluna
T_C=c_C*t_C;% Thickness coluna= chord*t

%Reynolds numbers
Re_LF=(rho)*(speed_LF)*(c_FF)/(mu); %Num Reynolds foil frente
Re_RF=(rho)*(speed_RF)*(c_FF)/(mu); %Num Reynolds foil frente
Re_ReF=(rho)*(speed_ReF)*(c_ReF)/(mu); %Num Reynold foil tras
Re_LS=(rho)*(speed_LS)*(c_S)/(mu); %Num Reynolds strut
Re_RS=(rho)*(speed_RS)*(c_S)/(mu); %Num Reynolds strut
Re_C=(rho)*(speed_C)*(c_C)/(mu); %Num Reynolds coluna

%% Determining cd of the foils, struts and prop column

%strut pressure drag. Column assumed to have same pressure drag as
%strut
p00 =     0.01162;
p10 =  -7.938e-07;
p01 =  -5.664e-05;
p20 =   0.0001378;
p11 =   3.735e-08;
p02 =   1.241e-07;
p30 =  -1.257e-07;
p21 =   -4.13e-07;
p12 =  -9.269e-11;
p03 =  -1.231e-10;
p40 =   1.604e-06;
p31 =    4.88e-10;
p22 =   4.056e-10;
p13 =   6.432e-14;
p04 =   5.515e-14;
p50 =  -1.201e-09;
p41 =  -1.096e-09;
p32 =   -1.95e-13;
p23 =   -1.04e-13;
p14 =   -1.36e-17;
p05 =   -9.13e-18;

cdp_S =@(x,y) p00 + p10*x + p01*y + p20*x^2 + p11*x*y + p02*y^2 + p30*x^3 + p21*x^2*y ...
    + p12*x*y^2 + p03*y^3 + p40*x^4 + p31*x^3*y + p22*x^2*y^2 ...
    + p13*x*y^3 + p04*y^4 + p50*x^5 + p41*x^4*y + p32*x^3*y^2 ...
    + p23*x^2*y^3 + p14*x*y^4 + p05*y^5;

CDp_LS = cdp_S(bb_LS,Re_LS/1000);
CDp_RS = cdp_S(bb_RS,Re_RS/1000);
CDp_C = cdp_S(bb_C+Rudder,Re_C/1000);

%determining coefficient of lift of the foils for a set angle of attack
p00 =     0.04647;
p10 =      0.1369;
p01 =    0.001502;
p20 =   0.0005872;
p11 =  -0.0001138;
p02 =  -2.794e-06;
p30 =  -0.0007229;
p21 =  -2.662e-07;
p12 =   1.545e-07;
p03 =   2.428e-09;
p40 =   1.647e-05;
p31 =   6.574e-07;
p22 =  -3.892e-09;
p13 =  -7.221e-11;
p04 =  -9.966e-13;
p50 =  -6.807e-08;
p41 =  -2.534e-09;
p32 =  -2.657e-10;
p23 =   2.267e-12;
p14 =   9.751e-15;
p05 =   1.555e-16;

cl = @(x,y) p00 + p10*x + p01*y + p20*x^2 + p11*x*y + p02*y^2 + p30*x^3 + p21*x^2*y ...
    + p12*x*y^2 + p03*y^3 + p40*x^4 + p31*x^3*y + p22*x^2*y^2 ...
    + p13*x*y^3 + p04*y^4 + p50*x^5 + p41*x^4*y + p32*x^3*y^2 ...
    + p23*x^2*y^3 + p14*x*y^4 + p05*y^5;

cl_LF = cl(eff_aa_LF,Re_LF/1000);
cl_RF = cl(eff_aa_RF,Re_RF/1000);
cl_ReF = cl(eff_aa_ReF,Re_ReF/1000);
CL_3D_LF =cl_LF*(AR_FF/(AR_FF+2))*k2_LF;
CL_3D_RF =cl_RF*(AR_FF/(AR_FF+2))*k2_RF;
CL_3D_ReF =cl_ReF*(AR_ReF/(AR_ReF+2))*k2_ReF;

%determining coefficient of pressure drag of the foils
p00 =     0.01465;
p10 =  -0.0003439;
p01 =  -5.436e-05;
p20 =  -0.0002518;
p11 =   1.629e-06;
p02 =   8.999e-08;
p30 =   1.962e-05;
p21 =   5.111e-07;
p12 =  -2.115e-09;
p03 =  -7.446e-11;
p40 =    6.85e-06;
p31 =  -4.153e-08;
p22 =  -2.604e-10;
p13 =   1.213e-12;
p04 =   3.002e-14;
p50 =  -3.572e-07;
p41 =  -2.379e-09;
p32 =   1.914e-11;
p23 =   3.918e-14;
p14 =  -2.599e-16;
p05 =  -4.682e-18;

cdpf = @(x,y) p00 + p10*x + p01*y + p20*x^2 + p11*x*y + p02*y^2 + p30*x^3 + p21*x^2*y ...
    + p12*x*y^2 + p03*y^3 + p40*x^4 + p31*x^3*y + p22*x^2*y^2 ...
    + p13*x*y^3 + p04*y^4 + p50*x^5 + p41*x^4*y + p32*x^3*y^2 ...
    + p23*x^2*y^3 + p14*x*y^4 + p05*y^5;

cdp_LF = cdpf(eff_aa_LF,Re_LF/1000);
cdp_RF = cdpf(eff_aa_RF,Re_RF/1000);
cdp_ReF = cdpf(eff_aa_ReF,Re_ReF/1000);

%%%%%%%%%%%%%%%%%%%%%%%%%%%%%%%%%%%%%%%%%%%%%%%%%
%%%%%%%%%%%% boat model equations %%%%%%%%%%%%%%%
%%%%%%%%%%%%%%%%%%%%%%%%%%%%%%%%%%%%%%%%%%%%%%%%%

%Lift (XFRL5)
L_LF=(CL_3D_LF)*q_LF*S_FF;
L_RF=(CL_3D_RF)*q_RF*S_FF;
L_ReF=(CL_3D_ReF)*q_ReF*S_ReF;

k_LS=1/(13+(13/(sub_LS)^2)+(26/(sub_LS))); % coeficiente de lift que toma em conta a aspect ratio da seccao submergida da strut
k_RS=1/(13+(13/(sub_RS)^2)+(26/(sub_RS))); % coeficiente de lift que toma em conta a aspect ratio da seccao submergida da strut
k_C=1/(13+(13/(sub_C)^2)+(26/(sub_C))); % coeficiente de lift que toma em conta a aspect ratio da seccao submergida da coluna
L_LS = -1/2*rho*(speed_LS^2)*S_LS*k_LS*bb_LS;
L_RS = -1/2*rho*(speed_RS^2)*S_RS*k_RS*bb_RS;
L_C = -1/2*rho*(speed_C^2)*S_C*k_C*(bb_C+Rudder);
bb_Trans_sup = 12;
bb_Trans_inf = 15;

% condicão de ventilacão da strut esquerda
if bb_LS>bb_Trans_sup || bb_LS<-bb_Trans_sup 
    Lift_Trans_sup_LS = -1/2*rho*(speed_LS^2)*S_LS*k_LS*bb_Trans_sup*bb_LS/abs(bb_LS);
    Lift_Trans_inf_LS = -1/2*rho*(speed_LS^2)*S_LS*(k_LS*bb_Trans_inf*bb_LS/abs(bb_LS)-k_LS*9*(bb_LS/abs(bb_LS))*abs(1-abs(1/bb_Trans_inf)));
    L_LS = Lift_Trans_sup_LS+(Lift_Trans_inf_LS-Lift_Trans_sup_LS)/(bb_Trans_inf*bb_LS/abs(bb_LS)-bb_Trans_sup*bb_LS/abs(bb_LS))*(bb_LS-bb_Trans_sup*bb_LS/abs(bb_LS));
    if bb_LS>bb_Trans_inf || bb_LS<-bb_Trans_inf
        L_LS = -1/2*rho*(speed_LS^2)*S_LS*(k_LS*bb_LS-k_LS*9*(bb_LS/abs(bb_LS))*abs(1-abs(1/bb_LS)));      
    end
end
% condicão de ventilacão da strut direita
if bb_RS>bb_Trans_sup || bb_RS<-bb_Trans_sup 
    Lift_Trans_sup_RS = -1/2*rho*(speed_RS^2)*S_RS*k_RS*bb_Trans_sup*bb_RS/abs(bb_RS);
    Lift_Trans_inf_RS = -1/2*rho*(speed_RS^2)*S_RS*(k_RS*bb_Trans_inf*bb_RS/abs(bb_RS)-k_RS*9*(bb_RS/abs(bb_RS))*abs(1-abs(1/bb_Trans_inf)));
    L_RS = Lift_Trans_sup_RS+(Lift_Trans_inf_RS-Lift_Trans_sup_RS)/(bb_Trans_inf*bb_RS/abs(bb_RS)-bb_Trans_sup*bb_RS/abs(bb_RS))*(bb_RS-bb_Trans_sup*bb_RS/abs(bb_RS));
    if bb_RS>bb_Trans_inf || bb_RS<-bb_Trans_inf
        L_RS = -1/2*rho*(speed_RS^2)*S_RS*(k_RS*bb_RS-k_RS*9*(bb_RS/abs(bb_RS))*abs(1-abs(1/bb_RS)));
    end
end
% condicão de ventilacão da coluna
if (bb_C+Rudder)>bb_Trans_sup || (bb_C+Rudder)<-bb_Trans_sup
    Lift_Trans_sup_C = -1/2*rho*speed_C^2*S_C*k_C*bb_Trans_sup*(bb_C+Rudder)/abs(bb_C+Rudder);
    Lift_Trans_inf_C = -1/2*rho*speed_C^2*S_C*(k_C*bb_Trans_inf*(bb_C+Rudder)/abs(bb_C+Rudder)-k_C*9*(bb_C+Rudder)/abs(bb_C+Rudder));
    L_C = Lift_Trans_sup_C+(Lift_Trans_inf_C-Lift_Trans_sup_C)/(bb_Trans_inf*(bb_C+Rudder)/abs(bb_C+Rudder)-bb_Trans_sup*(bb_C+Rudder)/abs(bb_C+Rudder))*((bb_C+Rudder)-bb_Trans_sup*(bb_C+Rudder)/abs(bb_C+Rudder));
    if bb_C>bb_Trans_inf || bb_C<-bb_Trans_inf
        L_C = -1/2*rho*speed_C^2*S_C*(k_C*(bb_C+Rudder)-k_C*9*(bb_C+Rudder)/abs(bb_C+Rudder));
    end
end

%Induced Drag (XFLR5)
e=1; %oswald efficiency factor (assumir 1 para dist. lift puramente eliptica)
C_Dind_LF=(CL_3D_LF)^2/(pi*e*(AR_FF)); % Coef Drag Induzido
C_Dind_RF=(CL_3D_RF)^2/(pi*e*(AR_FF)); % Coef Drag Induzido
C_Dind_ReF=(CL_3D_ReF)^2/(pi*e*(AR_ReF));
D_induced_LF=(C_Dind_LF)*q_LF*(S_FF); %Drag induzido (N)
D_induced_RF=(C_Dind_RF)*q_RF*(S_FF); %Drag induzido (N)
D_induced_ReF=(C_Dind_ReF)*q_ReF*(S_ReF); %Drag induzido (N)

% Skin Friction Drag

Re_crit=500000;  %Como Rule Of Thumb, assume-se que a transição se dá pontualemente a Re=500 000- Anderson's Fundamentals of Aerodynamics (pg 903)
x_crit_LF=Re_crit*mu/(rho*speed_LF); %calcula o ponto onde se dá a transição na asa retângular
x_crit_RF=Re_crit*mu/(rho*speed_RF);
x_crit_ReF=Re_crit*mu/(rho*speed_ReF);
x_crit_LS=Re_crit*mu/(rho*speed_LS);
x_crit_RS=Re_crit*mu/(rho*speed_RS);
x_crit_C=Re_crit*mu/(rho*speed_C);
%x_c_crit_n63412=; %  <-M
%x_c_crit_n0012=0.3; %     <-M
%VARIAVEIS DE INPUT VAZIAS PARA FORÇAR A
%TRANSIÇAO NUM PONTO QUE NAO RE 500 000

%Left foil

C_skf_ff_lam=1.328/(Re_crit)^0.5; %Coef skin friction esc laminar- Hoerner’s Fluid-Dynamic Drag (pg 2-5)-Foil frente
S_ff_lam=S_FF*x_crit_LF; %Area de escoamento laminar- corresponde a zona 1-lam
D_skf_ff_lam=q_LF*C_skf_ff_lam*S_ff_lam; %Drag skf foil frente_flat plate_zona 1-lam
C_skf_ff_tur_12=0.455/(log10(Re_LF)^2.58); %Coef skin friction esc turbulento- Hoerner’s Fluid-Dynamic Drag (pg 2-5)-fim zona 2-tur
C_skf_ff_tur_1=0.455/(log10(Re_crit)^2.58); %coef skf ff esc turbulento- fim zona 1-trans
D_skf_ff_tur_12=q_LF*S_FF*C_skf_ff_tur_12; %drag skf ff_flat plate_esc turbulento-fim zona 2-tur
D_skf_ff_tur_1=q_LF*S_ff_lam*C_skf_ff_tur_1;%drag skf ff_flat plate_esc turbulento- fim zona 1-trans
D_skf_ff_tur=D_skf_ff_tur_12-D_skf_ff_tur_1;%drag skf ff_flat plate_esc turbulento total
D_skf_ff_tot_1=D_skf_ff_lam +D_skf_ff_tur; %drag skf ff_flat plate_total
CD_skf_ff=D_skf_ff_tot_1/(q_LF*S_FF); %coeficiente de drag de skin friction ff final
D_skf_LF=1/2*(CD_skf_ff)*(rho)*(speed_LF)^2*(SA_FF); %Drag de skin friction final ff

%Right foil
C_skf_ff_lam=1.328/(Re_crit)^0.5; %Coef skin friction esc laminar- Hoerner’s Fluid-Dynamic Drag (pg 2-5)-Foil frente
S_ff_lam=S_FF*x_crit_RF; %Area de escoamento laminar- corresponde a zona 1-lam
D_skf_ff_lam=q_RF*C_skf_ff_lam*S_ff_lam; %Drag skf foil frente_flat plate_zona 1-lam
C_skf_ff_tur_12=0.455/(log10(Re_RF)^2.58); %Coef skin friction esc turbulento- Hoerner’s Fluid-Dynamic Drag (pg 2-5)-fim zona 2-tur
C_skf_ff_tur_1=0.455/(log10(Re_crit)^2.58); %coef skf ff esc turbulento- fim zona 1-trans
D_skf_ff_tur_12=q_RF*S_FF*C_skf_ff_tur_12; %drag skf ff_flat plate_esc turbulento-fim zona 2-tur
D_skf_ff_tur_1=q_RF*S_ff_lam*C_skf_ff_tur_1;%drag skf ff_flat plate_esc turbulento- fim zona 1-trans
D_skf_ff_tur=D_skf_ff_tur_12-D_skf_ff_tur_1;%drag skf ff_flat plate_esc turbulento total
D_skf_ff_tot_1=D_skf_ff_lam +D_skf_ff_tur; %drag skf ff_flat plate_total
CD_skf_ff=D_skf_ff_tot_1/(q_RF*S_FF); %coeficiente de drag de skin friction ff final
D_skf_RF=1/2*(CD_skf_ff)*(rho)*(speed_RF)^2*(SA_FF); %Drag de skin friction final ff

%Rear foil
C_skf_ft_lam=1.328/(Re_crit)^0.5;%Coef skin friction esc laminar- Hoerner’s Fluid-Dynamic Drag (pg 2-5)-Foil tras
S_ft_lam=S_ReF*x_crit_ReF; %Area de escoamento laminar- corresponde a zona 1-lam
D_skf_ft_lam=q_ReF*C_skf_ft_lam*S_ft_lam;%Drag skf foil tras_flat plate_zona 1-lam
C_skf_ft_tur_12=0.455/(log10(Re_ReF)^2.58); %Coef skin friction esc turbulento- Hoerner’s Fluid-Dynamic Drag (pg 2-5)-fim zona 2-tur
C_skf_ft_tur_1=0.455/(log10(Re_crit)^2.58); %coef skf ft esc turbulento- fim zona 1-trans
D_skf_ft_tur_12=q_ReF*S_ReF*C_skf_ft_tur_12;%drag skf ft_flat plate_esc turbulento-fim zona 2-tur
D_skf_ft_tur_1=q_ReF*S_ft_lam*C_skf_ft_tur_1;%drag skf ft_flat plate_esc turbulento- fim zona 1-trans
D_skf_ft_tur=D_skf_ft_tur_12-D_skf_ft_tur_1;%drag skf ft_flat plate_esc turbulento total
D_skf_ft_tot_1=D_skf_ft_lam +D_skf_ft_tur; %drag skf ft_flat plate_total
CD_skf_ft=D_skf_ft_tot_1/(q_ReF*S_ReF);%coeficiente de drag de skin friction ft final
D_ftskt=1/2*(CD_skf_ft)*(rho)*(speed_ReF)^2*(SA_ReF);%Drag de skin friction final ft



%Strut Esquerda
C_skf_s_lam=1.328/(Re_crit)^0.5;%Coef skin friction esc laminar- Hoerner’s Fluid-Dynamic Drag (pg 2-5)-strut
S_s_lam_left=S_LS*x_crit_LS; %Area de escoamento laminar- corresponde a zona 1-lam
D_skf_s_lam_left=q_LS*C_skf_s_lam*S_s_lam_left;%Drag skf strut_flat plate_zona 1-lam
C_skf_s_tur_12=0.455/(log10(Re_LS)^2.58);%Coef skin friction esc turbulento- Hoerner’s Fluid-Dynamic Drag (pg 2-5)-fim zona 2-tur
C_skf_s_tur_1=0.455/(log10(Re_crit)^2.58);%coef skf s esc turbulento- fim zona 1-trans
D_skf_s_tur_12_left=q_LS*S_LS*C_skf_s_tur_12;%drag skf s_flat plate_esc turbulento-fim zona 2-tur
D_skf_s_tur_1_left=q_LS*S_s_lam_left*C_skf_s_tur_1;%drag skf s_flat plate_esc turbulento- fim zona 1-trans
D_skf_s_tur_left=D_skf_s_tur_12_left-D_skf_s_tur_1_left; %drag skf s_flat plate_esc turbulento total
D_skf_s_tot_1_left=D_skf_s_lam_left +D_skf_s_tur_left; %drag skf s_flat plate_total
CD_skf_s_left=D_skf_s_tot_1_left/(q_LS*S_LS);%coeficiente de drag de skin friction s final
D_strutskf_left=1/2*(CD_skf_s_left)*(rho)*(speed_LS)^2*(SA_LS);%Drag de skin friction final strut

%Strut Direita
C_skf_s_lam=1.328/(Re_crit)^0.5;%Coef skin friction esc laminar- Hoerner’s Fluid-Dynamic Drag (pg 2-5)-strut
S_s_lam_right=S_RS*x_crit_RS; %Area de escoamento laminar- corresponde a zona 1-lam
D_skf_s_lam_right=q_RS*C_skf_s_lam*S_s_lam_right;%Drag skf strut_flat plate_zona 1-lam
C_skf_s_tur_12=0.455/(log10(Re_RS)^2.58);%Coef skin friction esc turbulento- Hoerner’s Fluid-Dynamic Drag (pg 2-5)-fim zona 2-tur
C_skf_s_tur_1=0.455/(log10(Re_crit)^2.58);%coef skf s esc turbulento- fim zona 1-trans
D_skf_s_tur_12_right=q_RS*S_RS*C_skf_s_tur_12;%drag skf s_flat plate_esc turbulento-fim zona 2-tur
D_skf_s_tur_1_right=q_RS*S_s_lam_right*C_skf_s_tur_1;%drag skf s_flat plate_esc turbulento- fim zona 1-trans
D_skf_s_tur_right=D_skf_s_tur_12_right-D_skf_s_tur_1_right; %drag skf s_flat plate_esc turbulento total
D_skf_s_tot_1_right=D_skf_s_lam_right +D_skf_s_tur_right; %drag skf s_flat plate_total
CD_skf_s_right=D_skf_s_tot_1_right/(q_RS*S_RS);%coeficiente de drag de skin friction s final
D_strutskf_right=1/2*(CD_skf_s_right)*(rho)*(speed_RS)^2*(SA_RS);%Drag de skin friction final strut


%Column
C_skf_c_lam=1.328/(Re_crit)^0.5;%Coef skin friction esc laminar- Hoerner’s Fluid-Dynamic Drag (pg 2-5)-coluna
S_c_lam=S_C*x_crit_C;%Area de escoamento laminar- corresponde a zona 1-lam
D_skf_c_lam=q_C*C_skf_c_lam*S_c_lam;%Drag skf coluna_flat plate_zona 1-lam
C_skf_c_tur_lt=0.455/(log10(Re_C)^2.58);%Coef skin friction esc turbulento- Hoerner’s Fluid-Dynamic Drag (pg 2-5)-fim zona 2-tur
C_skf_c_tur_l=0.455/(log10(Re_crit)^2.58);%coef skf c esc turbulento- fim zona 1-trans
D_skf_c_tur_lt=q_C*S_C*C_skf_c_tur_lt;%drag skf c_flat plate_esc turbulento-fim zona 2-tur
D_skf_c_tur_l=q_C*S_c_lam*C_skf_c_tur_l;%drag skf c_flat plate_esc turbulento- fim zona 1-trans
D_skf_c_tur=D_skf_c_tur_lt-D_skf_c_tur_l;%drag skf c_flat plate_esc turbulento total
D_skf_c_tot_1=D_skf_c_lam +D_skf_c_tur;%drag skf c_flat plate_total
CD_skf_c=D_skf_c_tot_1/(q_C*S_C);%coeficiente de drag de skin friction c final
D_skfc=1/2*(CD_skf_c)*(rho)*(speed_C)^2*(SA_C); %Drag de skin friction final coluna

%Form Drag
D_form_LF_left=(cdp_LF)*q_LF*(S_FF);
D_form_RF_right=(cdp_RF)*q_RF*(S_FF);
D_form_ReF=(cdp_ReF)*q_ReF*(S_ReF);
D_form_LS=(CDp_LS)*q_LS*(S_LS);
D_form_RS=(CDp_RS)*q_RS*(S_RS);
D_form_C=(CDp_C)*q_C*(2*S_C);

%Interference Drag
C_Dint_FF=17*(t_FF)^2-.05; %Coef Drag interferencia- Hoerner’s Fluid Dynamic Drag (pg 8-1)
C_Dint_ReF=17*(t_ReF)^2-.05; %Coef Drag interferencia- Hoerner’s Fluid Dynamic Drag (pg 8-1)
D_interference_LF=q_LF*(C_Dint_FF)*((T_FF+T_S)/2)^2;%Drag Interferencia (N)
D_interference_RF=q_RF*(C_Dint_FF)*((T_FF+T_S)/2)^2;%Drag Interferencia (N)
D_interference_ReF=q_ReF*(C_Dint_ReF)*((T_ReF+T_C)/2)^2;%Drag Interferencia (N)

%Spray Drag
F_h_LS= speed_LS/(g*h_LS)^(0.5);%Numero de Froude a profundidade da strut
F_h_RS= speed_RS/(g*h_RS)^(0.5);%Numero de Froude a profundidade da strut
F_h_C= speed_C/(g*h_C)^(0.5);%Numero de Froude a profundidade da coluna
%Froude numbers ~3<
CDs=0.24; %coeficiente empirico de spray @Hoerner_Fluid-Dynamic Drag (10-13)
Ds_LS=q_LS*CDs*(t_S*c_S)^2;%Drag de spray para uma strut
Ds_RS=q_RS*CDs*(t_S*c_S)^2;%Drag de spray para uma strut
Ds_C=q_ReF*CDs*(t_C*c_C)^2;%Drag de spray para a coluna

%Wave Drag
CDw_LF=0.5*(CL_3D_LF/(F_h_LS*2))^2;
CDw_RF=0.5*(CL_3D_RF/(F_h_RS*2))^2;
CDw_C=0.5*(CL_3D_ReF/(F_h_C*2))^2;
Dw_LF=q_LF*CDw_LF*h_LS*b_FF;
Dw_RF=q_RF*CDw_RF*h_RS*b_FF;
Dw_C=q_C*CDw_C*h_C*b_ReF;


%Total Drag

D_LF=D_induced_RF+D_skf_LF+D_form_RF_right+D_interference_LF+Dw_RF;
D_RF=D_induced_LF+D_skf_RF+D_form_LF_left+D_interference_RF+Dw_LF;
D_ReF=D_induced_ReF+D_ftskt+D_form_ReF+D_interference_ReF+Dw_C;
D_LS=D_strutskf_left+D_form_LS+Ds_LS;
D_RS=D_strutskf_right+D_form_RS+Ds_RS;
D_C=D_skfc+D_form_C+Ds_C;

%Hull
CD_H = 0.006;% CFD Data
zp = -z_cm*100;
if (zp < 32 + 5/22)
    Hull_area = -0.2167*zp+6.98365;
else
    Hull_area = 0;
end
D_H = 0.5*CD_H*rho*Hull_area*speed_cm^2;
V_HULL = 0.001*zp^2-0.064*zp+1.03025;
if (zp >= 31)
    V_HULL1 = 0.001*31^2-0.064*31+1.03025;
    V_HULL = V_HULL1 + (-V_HULL1)/(32+5/22-31)*(zp-31);
end
if zp >= 32+5/22
    V_HULL = 0;
end
BUOYANCY = V_HULL*rho*g;


%calculate Thrust based on rpms
Rpms_propeller = Rpms_motor/2.85;
diam = 0.25;

%Interpolation coefficients of thrust
p1 =     -0.2264;
p2 =      0.8165;
p3 =     -0.9315;
p4 =      0.2713;
p5 =   -0.009195;
p6 =   -0.005493;
p7 =      0.1617;

%Interpolation coefficients of proppeler's efficiency

k1 =      -170.6;
k2 =       30.69;
k3 =      -50.99;
k4 =       440.2;
k5 =      -1.744;
q1 =      -201.3;
q2 =       93.96;
q3 =       150.8;
q4 =      -151.9;
q5 =       398.2;

js = 60*speed_cm/(Rpms_propeller*diam);
ktfun = @(x) p1*x.^6 + p2*x.^5 + p3*x.^4 + p4*x.^3 + p5*x.^2 + p6*x + p7;

kt =ktfun(js);

Efffun = @(x)(k1*x.^4 + k2*x.^3 + k3*x.^2 + k4*x + k5) /...
    (x.^5 + q1*x.^4 + q2*x.^3 + q3*x.^2 + q4*x + q5);

Eff = Efffun(js);

Thrust = rho*(Rpms_propeller/60)^2*diam^4*kt;
P_propeller = Thrust*speed_cm/Eff;

%Calculate Power usage
P_mec=P_propeller/0.96;
Torque=P_mec/(Rpms_motor*2*pi/60);

%%%%%%%%%%%%%%%%%%%%%%%%%Balances of forces and momenta%%%%%%%%%%%%%%%%
%%%%%%%%%%%%%%%%%%%%%%%%%%%%%%%%%%%%%%%%%%%%%%%%%%%%%%%%%%%%%%%%%%%%%%%

%Inertial forces
W_inertial = m*g*[0;0;1];
BUOY_inertial = BUOYANCY*[0;0;-1];

%Body frame forces
L_b_LF = L_LF*[sind(aa_LF);0;-cosd(aa_LF)];
L_b_RF = L_RF*[sind(aa_RF);0;-cosd(aa_RF)];
L_b_ReF = L_ReF*[sind(aa_ReF);0;-cosd(aa_ReF)];
L_b_LS = L_LS*[-sind(bb_LS);cosd(bb_LS);0];
L_b_RS = L_RS*[-sind(bb_RS);cosd(bb_RS);0];
L_b_C = L_C*[-sind(bb_C);cosd(bb_C);0];
D_b_LF = D_LF*[-cosd(aa_LF);0;-sind(aa_LF)];
D_b_RF = D_RF*[-cosd(aa_RF);0;-sind(aa_RF)];
D_b_ReF = D_ReF*[-cosd(aa_ReF);0;-sind(aa_ReF)];
D_b_LS = D_LS*[-cosd(bb_LS);-sind(bb_LS);0];
D_b_RS = D_RS*[-cosd(bb_RS);-sind(bb_RS);0];
D_b_C = D_C*[-cosd(bb_C);-sind(bb_C);0];
D_b_H = D_H*[-u/speed_cm;-v/speed_cm;-w/speed_cm];

%Sum of body frame forces in each location to calculate momenta
X_LF = L_b_LF(1) + D_b_LF(1);
Y_LF = 0;
Z_LF = L_b_LF(3) + D_b_LF(3);
X_RF = L_b_RF(1) + D_b_RF(1);
Y_RF = 0;
Z_RF = L_b_RF(3) + D_b_RF(3);
X_ReF = L_b_ReF(1)+D_b_ReF(1);
Y_ReF =  0;
Z_ReF = L_b_ReF(3)+D_b_ReF(3);
X_LS = L_b_LS(1) + D_b_LS(1);
Y_LS = L_b_LS(2) + D_b_LS(2);
Z_LS = 0;
X_RS = L_b_RS(1) + D_b_RS(1);
Y_RS = L_b_RS(2) + D_b_RS(2);
Z_RS = 0;
X_C = L_b_C(1) + D_b_C(1);
Y_C = L_b_C(2) + D_b_C(2);
Z_C = 0;
Y_Prop = -Thrust*sind(Rudder);
X_Prop = Thrust*cosd(Rudder);

%Sum of body forces in body axis
X = X_LF + X_RF + X_ReF + X_LS + X_RS + X_C + X_Prop +  D_b_H(1);
Y = Y_LF + Y_RF + Y_ReF + Y_LS + Y_RS + Y_C + Y_Prop +  D_b_H(2);
Z = Z_LF + Z_RF + Z_ReF + Z_LS + Z_RS + Z_C + D_b_H(3);

F = [X;Y;Z];

%Sum of moments in body axis
M_np= CM_ac*(q_LF*S_FF*c_FF+q_RF*S_FF*c_FF+q_ReF*S_ReF*c_ReF); %neutral point moment (from wing AC moments)
L = -Y_LS*LS_CoP-Z_LF*dist_FF_cm_y-Y_RS*RS_CoP +Z_RF*dist_FF_cm_y-Y_C*C_CoP - Y_Prop*(dist_ReF_cm_z-0.2); %dist z of propeller 
M = X_LF*dist_FF_cm_z+X_LS*LS_CoP + X_RF*dist_FF_cm_z+X_RS*RS_CoP-Z_LF*dist_FF_cm_x-Z_RF*dist_FF_cm_x+Z_ReF*dist_C_cm_x+X_ReF*dist_ReF_cm_z+X_C*C_CoP+X_Prop*(dist_FF_cm_z)+M_np;
N = X_LF*dist_FF_cm_y+X_LS*dist_FF_cm_y-X_RF*dist_FF_cm_y-X_RS*dist_FF_cm_y+Y_LF*dist_FF_cm_x+Y_LS*dist_FF_cm_x+Y_RF*dist_FF_cm_x+Y_RS*dist_FF_cm_x-Y_ReF*dist_C_cm_x-Y_C*dist_C_cm_x-Y_Prop*dist_C_cm_x;

Tau = [L;M;N];

%Balance of forces
p = p*pi/180;
qq = qq*pi/180;
r = r*pi/180;
ww = [p;qq;r];

uvw_dot = (F + R*W_inertial + R*BUOY_inertial)/m - cross(ww, [u;v;w]);

VI_dot = R'*[u;v;w];

%Balance of moments

J = [Ixx 0 Ixz;
     0   Iyy 0;
     Ixz 0 Izz];
invJ = [-Izz/(Ixz^2 - Ixx*Izz),     0,  Ixz/(Ixz^2 - Ixx*Izz);
            0,                  1/Iyy,                      0;
       Ixz/(Ixz^2 - Ixx*Izz),     0,  -Ixx/(Ixz^2 - Ixx*Izz)];

wdot = invJ*(Tau - cross(ww,J*ww));

p_dot = wdot(1)*180/pi;
q_dot = wdot(2)*180/pi;
r_dot = wdot(3)*180/pi;

u_dot = uvw_dot(1);
v_dot = uvw_dot(2);
w_dot = uvw_dot(3);

Z_dot = VI_dot(3);

end

== matlab function lqr_model/Filter2/2nd order Butter1/MATLAB Function ==
  data: y input; u input; yfilt output; by2 parameter; ay2 parameter
function yfilt = filtit(y,u, by2, ay2)
b = by2;
a = ay2;
yfilt = 0;
for i=1:length(u)
   yfilt = yfilt + b(i)*u(i);
end

for i=2:length(y)+1
   yfilt = yfilt - a(i)*y(i-1); 
end

yfilt = yfilt/a(1);

end
